simulink model "example1_cs"  (R2018b)
settings: Solver=ode5  StartTime=0.0  StopTime=inf  FixedStep=1/20  RelTol=1e-3
PreLoadFcn:
  | mbxruntime.callbacks.PreLoadFcn(bdroot);
PostLoadFcn:
  | mbxruntime.callbacks.PostLoadFcn(bdroot);
InitFcn:
  | mbxruntime.callbacks.InitFcn(bdroot);
StartFcn:
  | mbxruntime.callbacks.StartFcn(bdroot);
StopFcn:
  | mbxruntime.callbacks.StopFcn(bdroot);
model workspace: external: MAT-File example1_cs_hws.mat (data not in the file)
undefined symbols (not defined in the file or in its folder): Broadcast, CameraTimestamp, Confidence, ConfidenceType, DiscIntNeverNeededParam, ErrorCode, Header, Height, Id, Id_SL_Info, InitImageOutputDir, Length, LidarTimestamp, PerceptionObstacle, PerceptionObstacle_SL_Info, PolygonPoint, PolygonPoint_SL_Info, Pose, Position, RadarTimestamp, S, SequenceNum, Theta, Timestamp, TimestampSec, TrackingTime, Type, Velocity, warningInitialVelocity, Waypoint, Waypoint_SL_Info, Width, X, x0, Y, Z
libraries: simulink x27, robotlib x15, PreScanSimulinkLibrary x14, simulink_extras x5, robotcorelib x2
(part 3 of 5)

== system example1_cs/Ford_Focus_Stationwagon_1 ==
  SELF_Ford_Focus_Stationwagon_1 : Inport  Tag=inport/SelfPort  OutDataTypeStr=Bus: PRESCAN_SELFSENSORDATA  PortDimensions=1  SampleTime=1/20  BusOutputAsStruct=on
  Path : S-Function  Tag=Path  LoadFcn=load('PrescanMotionData.mat')  FunctionName=sfun_Path  Parameters=uniqueID, pathUniqueID, timestep  SFunctionDeploymentMode=off  EnableBusSupport=off  mask(Path){uniqueID=232, pathUniqueID=457, timestep=1/20}
      mask prompts: uniqueID "Object Unique ID"; pathUniqueID "Path Unique ID"; timestep "MATLAB timestep:"
      mask help:
      | The path block outputs the position along a given trajectory.
      |
      | For more information, please click Help.
      mask Help: eval('openHelp(312)')
      mask Display: image(imread('Path.png'))
  SELF_Demux : Subsystem  Tag=demux/SelfPort  mask(PreScan Demux Block:){}
      mask help:
      | The SELF port shows (state) information of the actor itself. The outputs are position in the experiment's axis system and the GPS coordinates, and the object's absolute velocity and compass heading.
      |
      | For more information, please click Help.
      settings: DeleteFcn=PreScanBlockDeleteFcn;
      mask Help: eval('openHelp(462)')
      mask Display:
      | port_label('output',1,'x [m]')
      | port_label('output',2,'y [m]')
      | port_label('output',3,'z [m]','texmode','on')
      | port_label('output',4,'Rotx [deg]','texmode','on')
      | port_label('output',5,'Roty [deg]','texmode','on')
      | port_label('output',6,'Rotz [deg]','texmode','on')
      | port_label('output',7,'GPS lat [deg]','texmode','on')
      | port_label('output',8,'GPS long [deg]','texmode','on')
      | port_label('output',9,'GPS alt [m]','texmode','on')
      | port_label('output',10,'Velocity [m/s]')
      | port_label('output',11,'Heading [deg]')
      | port_label('output',12,'Yaw rate [deg/s]')
  STATE_Ford_Focus_Stationwagon_1_rc : RateTransition  Tag=mux_rc/StatePort  OutPortSampleTimeOpt=Inherit
  SpeedProfile : S-Function  Tag=SpeedProfile  LoadFcn=load('PrescanMotionData.mat')  FunctionName=sfun_SpeedProfile  Parameters=speedProfileUniqueID, timestep  SFunctionDeploymentMode=off  EnableBusSupport=off  mask(SpeedProfile){speedProfileUniqueID=458, timestep=1/20}
      mask prompts: speedProfileUniqueID "Speed Profile Unique ID"; timestep "MATLAB timestep:"
      mask help:
      | The speed profile block outputs the travelled distance, velocities and acceleration along a given path.
      |
      | For more information, please click Help.
      mask Help: eval('openHelp(312)')
      mask Display: image(imread('SpeedProfile.png'))
  Terminator_{1..12} (12 alike) : Terminator
  STATE_Ford_Focus_Stationwagon_1_bus : Outport  Tag=outport/StatePort  OutDataTypeStr=Bus: PRESCAN_STATEACTUATORDATA  PortDimensions=1  SampleTime=1/20
  wires:
  STATE_Ford_Focus_Stationwagon_1_rc/1 -> STATE_Ford_Focus_Stationwagon_1_bus/1
  SpeedProfile/1 -> Path/1
  Path/1 -> STATE_Ford_Focus_Stationwagon_1_rc/1
  SELF_Ford_Focus_Stationwagon_1/1 -> SELF_Demux/1(SELF)
  SELF_Demux/1(x [m]) -> Terminator_1/1
  SELF_Demux/2(y [m]) -> Terminator_2/1
  SELF_Demux/3(z [m]) -> Terminator_3/1
  SELF_Demux/4(rotx [deg]) -> Terminator_4/1
  SELF_Demux/5(roty [deg]) -> Terminator_5/1
  SELF_Demux/6(rotz [deg]) -> Terminator_6/1
  SELF_Demux/7(GPS lat [deg]) -> Terminator_7/1
  SELF_Demux/8(GPS long [deg]) -> Terminator_8/1
  SELF_Demux/9(GPS alt [m]) -> Terminator_9/1
  SELF_Demux/10(velocity [m/s]) -> Terminator_10/1
  SELF_Demux/11(heading [deg]) -> Terminator_11/1
  SELF_Demux/12(yaw rate [deg/s]) -> Terminator_12/1

== system example1_cs/ObjectCameraSensor_1 ==
  Sensor : S-Function  FunctionName=sfun_OCS  Parameters=sensorID, detectableObjects, dataWidth, dataHeight, channelsPerImage, timestep  SFunctionDeploymentMode=off  EnableBusSupport=off  mask(PreScan Source Block: Object Camera Sensor){sensorID=68, detectableObjects=1, dataWidth=240, dataHeight=960, channelsPerImage=3, timestep=1/20}
      mask prompts: sensorID "Sensor ID"; detectableObjects "Max detectable objects:"; dataWidth "Data width"; dataHeight "Data Height"; channelsPerImage "Channels per image"; timestep "MATLAB timestep:"
      mask help: The Object Camera Sensor provides information on objects locations.
      mask Help: eval('openHelp(2401)')
      mask Display: image(imread('ObjectCameraSensorSL.png'))
  ObjectCameraSensor_1 : Outport  Tag=outport/ObjectCamera/data  OutDataTypeStr=Bus: PRESCAN_OCS_MESSAGE  PortDimensions=1  SampleTime=1/20
  ObjectCameraSensor_1_Image : Outport  Tag=outport/ObjectCamera/image  Port=2  OutDataTypeStr=uint8  SampleTime=1/20
  wires:
  Sensor/1 -> ObjectCameraSensor_1/1
  Sensor/2 -> ObjectCameraSensor_1_Image/1

== system example1_cs/PointCloudSensor_1 ==
  Sensor : S-Function  FunctionName=sfun_PCS  Parameters=sensorID, dataWidth, dataHeight, numChannels, dataType, timestep  SFunctionDeploymentMode=off  EnableBusSupport=off  mask(PreScan Source Block: Point Cloud Sensor){sensorID=260, dataWidth=160, dataHeight=960, numChannels=3, dataType=0, timestep=1/20}
      mask prompts: sensorID "Sensor ID"; dataWidth "Data Width"; dataHeight "Data Height"; numChannels "Channel Count"; dataType "Data Type"; timestep "MATLAB timestep:"
      mask help: The Point Cloud Sensor provides XYZ positions relative to the sensor
      mask Help: eval('openHelp(6400)')
      mask Display: image(imread('PointCloudSensorSL.png'))
  PointCloudSensor_1 : Outport  Tag=outport/PointCloudInport  OutDataTypeStr=single  SampleTime=1/20
  wires:
  Sensor/1 -> PointCloudSensor_1/1

== system example1_cs/PreScanTerminator ==
  Terminator : Terminator
  sfun_Terminator : S-Function  FunctionName=sfun_Terminator  Parameters=SampleTime  SFunctionDeploymentMode=off  EnableBusSupport=off  mask(Legacy Function){SFunctionSpec=void prescan_terminator_outputFcn(void ** work1, PRESCAN_TERMINATORDATA y1[1]), SampleTime=TimeStep, ShowSpec=on}
      mask prompts: SampleTime "Sample time (-1 for inherited):"; ShowSpec "Display function specification"
      mask help:
      | This block allows you to call the legacy functions specified by the following Legacy Code Tool definition:
      | def.SFunctionName = 'sfun_Terminator';
      | def.OutputFcnSpec = 'void prescan_terminator_outputFcn(void ** work1, PRESCAN_TERMINATORDATA y1[1])';
      | def.StartFcnSpec = 'void prescan_terminator_startFcn(void ** work1)';
      | def.TerminateFcnSpec = 'void prescan_terminator_terminateFcn(void ** work1)';
      | def.HeaderFiles = {'prescan_terminator_data.h'};
      | def.HostLibFiles = {'sensorinterfaced.lib'};
      | def.IncPaths = {'src', 'C:\prescandev\vislibrary\vis\..\pimp\include\sensors\InterfaceRTW'};
      | def.SrcPaths = {'src'};
      | def.LibPaths = {'C:\\prescandev\\vislibrary_build\lib'};
      | def.SampleTime = 'parameterized';
      | def.Options.language = 'C';
      mask Help: <p>This block was generated automatically by the Legacy Code Tool. For detailed help on this tool, call<a href="matlab:legacy_code('help')"> legacy_code('help')</a>.</p>
      mask Callback ShowSpec:
      | if strcmp(get_param(gcbh, 'ShowSpec'), 'on')
      |   set_param(gcbh, 'MaskDisplay', sprintf('fprintf(''%s'');', get_param(gcbh, 'SFunctionSpec')));
      | else
      |   set_param(gcbh, 'MaskDisplay', sprintf('fprintf(''%s'');', get_param(gcbh, 'FunctionName')));
      | end
      mask Display: fprintf('void prescan_terminator_outputFcn(void ** work1, PRESCAN_TERMINATORDATA y1[1])');
  wires:
  sfun_Terminator/1 -> Terminator/1

== system example1_cs/SELF_BMW_X5_SUV_1 ==
  Sensor : S-Function  FunctionName=sfun_SelfSensor  Parameters=UniqueID, TimeStep  SFunctionDeploymentMode=off  EnableBusSupport=off  mask(PreScan Source Block: SELF){UniqueID=35, TimeStep=1/20}
      mask prompts: UniqueID "Auto-Assigned: Unique ID"; TimeStep "Auto-Assigned: Upload Period [s]"
      mask help:
      | The SELF port shows (state) information of the actor itself. The outputs are position in the experiment's axis system and the GPS coordinates, and the object's absolute velocity and compass heading.
      |
      | For more information, please click Help.
      mask Help: eval('openHelp(462)')
      mask Display: image(imread('GPS.png'))
  SELF_BMW_X5_SUV_1 : Outport  Tag=outport/SelfPort  OutDataTypeStr=Bus: PRESCAN_SELFSENSORDATA  PortDimensions=1  SampleTime=1/20
  wires:
  Sensor/1 -> SELF_BMW_X5_SUV_1/1

== system example1_cs/SELF_Boy_150_1 ==
  Sensor : S-Function  FunctionName=sfun_SelfSensor  Parameters=UniqueID, TimeStep  SFunctionDeploymentMode=off  EnableBusSupport=off  mask(PreScan Source Block: SELF){UniqueID=120, TimeStep=1/20}
      mask prompts: UniqueID "Auto-Assigned: Unique ID"; TimeStep "Auto-Assigned: Upload Period [s]"
      mask help:
      | The SELF port shows (state) information of the actor itself. The outputs are position in the experiment's axis system and the GPS coordinates, and the object's absolute velocity and compass heading.
      |
      | For more information, please click Help.
      mask Help: eval('openHelp(462)')
      mask Display: image(imread('GPS.png'))
  SELF_Boy_150_1 : Outport  Tag=outport/SelfPort  OutDataTypeStr=Bus: PRESCAN_SELFSENSORDATA  PortDimensions=1  SampleTime=1/20
  wires:
  Sensor/1 -> SELF_Boy_150_1/1

== system example1_cs/SELF_Ford_Focus_Stationwagon_1 ==
  Sensor : S-Function  FunctionName=sfun_SelfSensor  Parameters=UniqueID, TimeStep  SFunctionDeploymentMode=off  EnableBusSupport=off  mask(PreScan Source Block: SELF){UniqueID=232, TimeStep=1/20}
      mask prompts: UniqueID "Auto-Assigned: Unique ID"; TimeStep "Auto-Assigned: Upload Period [s]"
      mask help:
      | The SELF port shows (state) information of the actor itself. The outputs are position in the experiment's axis system and the GPS coordinates, and the object's absolute velocity and compass heading.
      |
      | For more information, please click Help.
      mask Help: eval('openHelp(462)')
      mask Display: image(imread('GPS.png'))
  SELF_Ford_Focus_Stationwagon_1 : Outport  Tag=outport/SelfPort  OutDataTypeStr=Bus: PRESCAN_SELFSENSORDATA  PortDimensions=1  SampleTime=1/20
  wires:
  Sensor/1 -> SELF_Ford_Focus_Stationwagon_1/1

== system example1_cs/STATE_BMW_X5_SUV_1_bus ==
  STATE_BMW_X5_SUV_1_bus : Inport  Tag=inport/StatePort  OutDataTypeStr=Bus: PRESCAN_STATEACTUATORDATA  PortDimensions=1  SampleTime=1/20  BusOutputAsStruct=on
  Actuator : S-Function  FunctionName=sfun_StateActuator  Parameters=UniqueID, TimeStep  SFunctionDeploymentMode=off  EnableBusSupport=off  mask(PreScan Sink Block: State){UniqueID=35, TimeStep=1/20}
      mask prompts: UniqueID "Auto-Assigned: Unique ID"; TimeStep "Auto-Assigned: Upload Period [s]"
      mask help:
      | The Actor State contains a vector signal of size (9x1), containing the following signals:
      |
      | -  Position    	(x,y,z)             	[m]
      | -  Velocity    	(vx,vy,vz)         	[m/s]
      | -  Angles       	(Roll, Pitch, Yaw)	[rad]
      |
      | The Actor state is defined in the global axis system.
      | The state is superponed on the Initial position defined in the GUI.
      |
      | For more information, please click Help.
      mask Help: eval('openHelp(222)')
      mask Display: image(imread('State.png'))
  wires:
  STATE_BMW_X5_SUV_1_bus/1 -> Actuator/1

== system example1_cs/STATE_Boy_150_1_bus ==
  STATE_Boy_150_1_bus : Inport  Tag=inport/StatePort  OutDataTypeStr=Bus: PRESCAN_STATEACTUATORDATA  PortDimensions=1  SampleTime=1/20  BusOutputAsStruct=on
  Actuator : S-Function  FunctionName=sfun_StateActuator  Parameters=UniqueID, TimeStep  SFunctionDeploymentMode=off  EnableBusSupport=off  mask(PreScan Sink Block: State){UniqueID=120, TimeStep=1/20}
      mask prompts: UniqueID "Auto-Assigned: Unique ID"; TimeStep "Auto-Assigned: Upload Period [s]"
      mask help:
      | The Actor State contains a vector signal of size (9x1), containing the following signals:
      |
      | -  Position    	(x,y,z)             	[m]
      | -  Velocity    	(vx,vy,vz)         	[m/s]
      | -  Angles       	(Roll, Pitch, Yaw)	[rad]
      |
      | The Actor state is defined in the global axis system.
      | The state is superponed on the Initial position defined in the GUI.
      |
      | For more information, please click Help.
      mask Help: eval('openHelp(222)')
      mask Display: image(imread('State.png'))
  wires:
  STATE_Boy_150_1_bus/1 -> Actuator/1

== system example1_cs/STATE_Ford_Focus_Stationwagon_1_bus ==
  STATE_Ford_Focus_Stationwagon_1_bus : Inport  Tag=inport/StatePort  OutDataTypeStr=Bus: PRESCAN_STATEACTUATORDATA  PortDimensions=1  SampleTime=1/20  BusOutputAsStruct=on
  Actuator : S-Function  FunctionName=sfun_StateActuator  Parameters=UniqueID, TimeStep  SFunctionDeploymentMode=off  EnableBusSupport=off  mask(PreScan Sink Block: State){UniqueID=232, TimeStep=1/20}
      mask prompts: UniqueID "Auto-Assigned: Unique ID"; TimeStep "Auto-Assigned: Upload Period [s]"
      mask help:
      | The Actor State contains a vector signal of size (9x1), containing the following signals:
      |
      | -  Position    	(x,y,z)             	[m]
      | -  Velocity    	(vx,vy,vz)         	[m/s]
      | -  Angles       	(Roll, Pitch, Yaw)	[rad]
      |
      | The Actor state is defined in the global axis system.
      | The state is superponed on the Initial position defined in the GUI.
      |
      | For more information, please click Help.
      mask Help: eval('openHelp(222)')
      mask Display: image(imread('State.png'))
  wires:
  STATE_Ford_Focus_Stationwagon_1_bus/1 -> Actuator/1

== system example1_cs/Synchronizer ==
  Bus Selector1 : BusSelector  OutputSignals=FederateStopped
  Stop Simulation : Stop
  sfun_Synchronizer : S-Function  FunctionName=sfun_Synchronizer  Parameters=SampleTime  SFunctionDeploymentMode=off  EnableBusSupport=off  mask(Legacy Function){SFunctionSpec=void prescan_synchronizer_outputFcn(void ** work1, PRESCAN_SYNCHRONIZEDATA y1[1]), SampleTime=TimeStep, ShowSpec=on}
      mask prompts: SampleTime "Sample time (-1 for inherited):"; ShowSpec "Display function specification"
      mask help:
      | This block allows you to call the legacy functions specified by the following Legacy Code Tool definition:
      | def.SFunctionName = 'sfun_Synchronizer';
      | def.OutputFcnSpec = 'void prescan_synchronizer_outputFcn(void ** work1, PRESCAN_SYNCHRONIZEDATA y1[1])';
      | def.StartFcnSpec = 'void prescan_synchronizer_startFcn(void ** work1)';
      | def.TerminateFcnSpec = 'void prescan_synchronizer_terminateFcn(void ** work1)';
      | def.HeaderFiles = {'prescan_synchronizer_data.h'};
      | def.HostLibFiles = {'sensorinterfaced.lib'};
      | def.IncPaths = {'src', 'C:\prescandev\vislibrary\vis\..\pimp\include\sensors\InterfaceRTW'};
      | def.SrcPaths = {'src'};
      | def.LibPaths = {'C:\\prescandev\\vislibrary_build\lib'};
      | def.SampleTime = 'parameterized';
      | def.Options.language = 'C';
      mask Help: <p>This block was generated automatically by the Legacy Code Tool. For detailed help on this tool, call<a href="matlab:legacy_code('help')"> legacy_code('help')</a>.</p>
      mask Callback ShowSpec:
      | if strcmp(get_param(gcbh, 'ShowSpec'), 'on')
      |   set_param(gcbh, 'MaskDisplay', sprintf('fprintf(''%s'');', get_param(gcbh, 'SFunctionSpec')));
      | else
      |   set_param(gcbh, 'MaskDisplay', sprintf('fprintf(''%s'');', get_param(gcbh, 'FunctionName')));
      | end
      mask Display: fprintf('void prescan_synchronizer_outputFcn(void ** work1, PRESCAN_SYNCHRONIZEDATA y1[1])');
  wires:
  Bus Selector1/1 -> Stop Simulation/1  "<FederateStopped>"
  sfun_Synchronizer/1 -> Bus Selector1/1

== system example1_cs/BMW_X5_SUV_1/BoundingRectangle_1_Demux ==
  BRS : Inport
  Bus Selector : BusSelector  OutputSignals=DATA.ObjectID,DATA.Left,DATA.Right,DATA.Bottom,DATA.Top
  For Iterator : ForIterator  ResetStates=reset  IterationLimit=detectableObjects
  Selector : Selector  InputPortWidth=detectableObjects  IndexOptions=Index vector (port)  Indices=[1 3]  OutputSizes=1
  Signal2ArrayOfSignals1 : Subsystem  mask{VECTORLENGTH=detectableObjects}
      mask prompts: VECTORLENGTH "Length of vector"
  Signal2ArrayOfSignals2 : Subsystem  mask{VECTORLENGTH=detectableObjects}
      mask prompts: VECTORLENGTH "Length of vector"
  Signal2ArrayOfSignals3 : Subsystem  mask{VECTORLENGTH=detectableObjects}
      mask prompts: VECTORLENGTH "Length of vector"
  Signal2ArrayOfSignals4 : Subsystem  mask{VECTORLENGTH=detectableObjects}
      mask prompts: VECTORLENGTH "Length of vector"
  Signal2ArrayOfSignals5 : Subsystem  mask{VECTORLENGTH=detectableObjects}
      mask prompts: VECTORLENGTH "Length of vector"
  ObjectID : Outport
  Left : Outport  Port=2
  Right : Outport  Port=3
  Bottom : Outport  Port=4
  Top : Outport  Port=5
  wires:
  Bus Selector/5 -> Signal2ArrayOfSignals5/2(Element)  "<Top>"
  Signal2ArrayOfSignals5/1(ArrayofElements) -> Top/1
  Bus Selector/4 -> Signal2ArrayOfSignals4/2(Element)  "<Bottom>"
  Signal2ArrayOfSignals4/1(ArrayofElements) -> Bottom/1
  Bus Selector/3 -> Signal2ArrayOfSignals3/2(Element)  "<Right>"
  Signal2ArrayOfSignals3/1(ArrayofElements) -> Right/1
  Bus Selector/2 -> Signal2ArrayOfSignals1/2(Element)  "<Left>"
  Signal2ArrayOfSignals1/1(ArrayofElements) -> Left/1
  Signal2ArrayOfSignals2/1(ArrayofElements) -> ObjectID/1
  Bus Selector/1 -> Signal2ArrayOfSignals2/2(Element)  "<ObjectID>"
  Selector/1 -> Bus Selector/1
  For Iterator/1 -> Signal2ArrayOfSignals4/1(LoopIndex), Signal2ArrayOfSignals5/1(LoopIndex), Signal2ArrayOfSignals3/1(LoopIndex), Signal2ArrayOfSignals1/1(LoopIndex), Signal2ArrayOfSignals2/1(LoopIndex), Selector/2
  BRS/1 -> Selector/1

== system example1_cs/BMW_X5_SUV_1/CameraSensor_1_CM_Demux ==
  In1 : Inport
  Selector : Selector  NumberOfDimensions=2  InputPortWidth=3  IndexOptions=Index vector (dialog),Index vector (dialog)  Indices=-1,1:hres  OutputSizes=1,1
  Selector1 : Selector  NumberOfDimensions=2  InputPortWidth=3  IndexOptions=Index vector (dialog),Index vector (dialog)  Indices=-1,hres+1:hres*2  OutputSizes=1,1
  Selector2 : Selector  NumberOfDimensions=2  InputPortWidth=3  IndexOptions=Index vector (dialog),Index vector (dialog)  Indices=-1,hres*2+1:hres*3  OutputSizes=1,1
  R : Outport
  G : Outport  Port=2
  B : Outport  Port=3
  wires:
  In1/1 -> Selector1/1, Selector/1, Selector2/1
  Selector/1 -> R/1
  Selector1/1 -> G/1
  Selector2/1 -> B/1

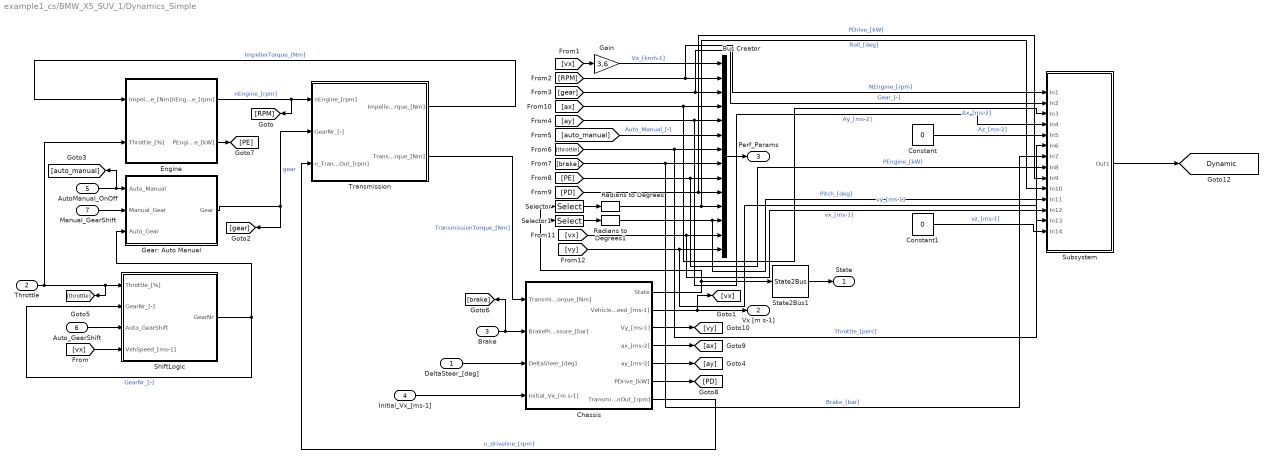
== system example1_cs/BMW_X5_SUV_1/Dynamics_Simple ==
  DeltaSteer_[deg] : Inport
  Throttle : Inport  Port=2
  Brake : Inport  Port=3
  Initial_Vx_[ms-1] : Inport  Port=4
  AutoManual_OnOff : Inport  Port=5
  Auto_GearShift : Inport  Port=6
  Manual_GearShift : Inport  Port=7
  Bus Creator : BusCreator  Inputs=14
  Chassis : Subsystem
      mask Display: image(imread('Chassis.png'));
  Constant : Constant  Value=0
  Constant1 : Constant  Value=0
  Engine : Subsystem
      mask Display: image(imread('Engine.png'));
  Gain : Gain  Gain=3.6
  Gear: Auto Manual : Subsystem
  Radians to Degrees : simulink_extras/Transformations/Radians to Degrees
  Radians to Degrees1 : simulink_extras/Transformations/Radians to Degrees
  Selector : Selector  InputPortWidth=9  IndexOptions=Index vector (dialog)  Indices=7  OutputSizes=1
  Selector1 : Selector  InputPortWidth=9  IndexOptions=Index vector (dialog)  Indices=8  OutputSizes=1
  ShiftLogic : Subsystem
      mask Display: image(imread('Gearshift.png'));
  State2Bus1 : PreScanSimulinkLibrary/State2Bus  Tag=State  Priority=0  x0=initialX  y0=initialY  z0=initialZ  Roll0=initialRoll  Pitch0=initialPitch  Yaw0=initialYaw  TimeStep=TimeStep
  Subsystem : Subsystem
  Transmission : Subsystem
      mask Display: image(imread('Transmission.png'));
  State : Outport
  Vx [m s-1] : Outport  Port=2
  Perf_Params : Outport  Port=3
  tag scope: Dynamic=global
  wires:
  State2Bus1/1 -> State/1
  [vy] -> Subsystem/13(In13), Bus Creator/14  "vy_[ms-1]"
  [vx] -> Subsystem/12(In12), Bus Creator/13  "vx_[ms-1]"
  Chassis/7(TransmissionOut_[rpm]) -> Transmission/3(n_TransmissionOut_[rpm])  "n_driveline_[rpm]"
  Chassis/6(PDrive_[kW]) -> [PD]
  Chassis/5(ay_[ms-2]) -> [ay]
  Chassis/4(ax_[ms-2]) -> [ax]
  Chassis/3(Vy_[ms-1]) -> [vy]
  [vx] -> ShiftLogic/4(VehSpeed_[ms-1])
  Gear: Auto Manual/1(Gear) -> Transmission/2(GearNr_[-]), [gear]  "gear"
  Manual_GearShift/1 -> Gear: Auto Manual/2(Manual_Gear)
  AutoManual_OnOff/1 -> Gear: Auto Manual/1(Auto_Manual), [auto_manual]
  Chassis/2(VehicleSpeed_[ms-1]) -> [vx], Vx [m s-1]/1
  Auto_GearShift/1 -> ShiftLogic/3(Auto_GearShift)
  Throttle/1 -> Engine/2(Throttle_[%]), ShiftLogic/1(Throttle_[%]), [throttle]
  Initial_Vx_[ms-1]/1 -> Chassis/4(Initial_Vx_[m s-1])
  DeltaSteer_[deg]/1 -> Chassis/3(DeltaSteer_[deg])
  Chassis/1(State) -> Selector/1, Selector1/1, State2Bus1/1
  Brake/1 -> [brake], Chassis/2(BrakePressure_[bar])
  Engine/1(nEngine_[rpm]) -> [RPM], Transmission/1(nEngine_[rpm])  "nEngine_[rpm]"
  ShiftLogic/1(GearNr) -> Gear: Auto Manual/3(Auto_Gear), ShiftLogic/2(GearNr_[-])  "GearNr_[-]"
  Transmission/2(TransmissionTorque_[Nm]) -> Chassis/1(TransmissionTorque_[Nm])  "TransmissionTorque_[Nm]"
  Transmission/1(ImpellerTorque_[Nm]) -> Engine/1(ImpellerTorque_[Nm])  "ImpellerTorque_[Nm]"
  Gain/1 -> Bus Creator/1  "Vx_[kmh-1]"
  [RPM] -> Subsystem/1(In1), Bus Creator/2  "NEngine_[rpm]"
  [gear] -> Subsystem/2(In2), Bus Creator/3  "Gear_[-]"
  [ay] -> Subsystem/4(In4), Bus Creator/5  "Ay_[ms-2]"
  [auto_manual] -> Bus Creator/6  "Auto_Manual_[-]"
  [throttle] -> Subsystem/6(In6), Bus Creator/7  "Throttle_[perc]"
  [brake] -> Subsystem/7(In7), Bus Creator/8  "Brake_[bar]"
  Engine/2(PEngine_[kW]) -> [PE]
  Bus Creator/1 -> Perf_Params/1
  [PE] -> Subsystem/8(In8), Bus Creator/9  "PEngine_[kW]"
  Radians to Degrees/1 -> Subsystem/10(In10), Bus Creator/11  "Roll_[deg]"
  Radians to Degrees1/1 -> Subsystem/11(In11), Bus Creator/12  "Pitch_[deg]"
  [PD] -> Subsystem/9(In9), Bus Creator/10  "PDrive_[kW]"
  Selector/1 -> Radians to Degrees/1
  Selector1/1 -> Radians to Degrees1/1
  [vx] -> Gain/1
  [ax] -> Subsystem/3(In3), Bus Creator/4  "Ax_[ms-2]"
  Constant/1 -> Subsystem/5(In5)  "Az_[ms-2]"
  Constant1/1 -> Subsystem/14(In14)  "vz_[ms-1]"
  Subsystem/1(Out1) -> [Dynamic]

== system example1_cs/BMW_X5_SUV_1/Enabled Subsystem ==
  In1 : Inport
  Enable : EnablePort
  Add : Sum
  Bus Selector : BusSelector  DialogController=Simulink.DDGSource_BusSelector  OutputSignals=Throttle,Brake,Debug.SimpleLatDebug.SteerAngle,Debug.SimpleLatDebug.RefSpeed,Debug.InputDebug.LocalizationHeader.TimestampSec
  Display : Display
  Ground_1 : Ground
  Product : Product
  Step : Step  Time=5  After=-30  SampleTime=0
  Step1 : Step  Time=5  Before=1  After=0  SampleTime=0
  Terminator_1 : Terminator
  Out1 : Outport
  Out2 : Outport  Port=2
  Out3 : Outport  Port=3
  Out5 : Outport  Port=4
  Out4 : Outport  Port=5
  wires:
  In1/1 -> Bus Selector/1
  Bus Selector/1 -> Out1/1  "<Throttle>"
  Bus Selector/2 -> Out2/1  "<Brake>"
  Bus Selector/4 -> Out5/1  "<RefSpeed>"
  Step/1 -> Add/1
  Step1/1 -> Product/2
  Product/1 -> Add/2
  Bus Selector/3 -> Out3/1, Display/1  "<SteerAngle>"
  Bus Selector/5 -> Out4/1  "<TimestampSec>"
  Add/1 -> Terminator_1/1
  Ground_1/1 -> Product/1

== system example1_cs/BMW_X5_SUV_1/Enabled Subsystem1 ==
  In1 : Inport
  Enable : EnablePort
  Add : Sum
  Bus Selector : BusSelector  DialogController=Simulink.DDGSource_BusSelector  OutputSignals=TrajectoryPoint,TrajectoryPoint_SL_Info
  Ground_1 : Ground
  Product : Product
  Step : Step  Time=5  After=-30  SampleTime=0
  Step1 : Step  Time=5  Before=1  After=0  SampleTime=0
  Terminator_1 : Terminator
  Out1 : Outport
  Out2 : Outport  Port=2
  wires:
  In1/1 -> Bus Selector/1
  Bus Selector/1 -> Out1/1  "<TrajectoryPoint>"
  Bus Selector/2 -> Out2/1  "<TrajectoryPoint_SL_Info>"
  Step/1 -> Add/1
  Step1/1 -> Product/2
  Product/1 -> Add/2
  Add/1 -> Terminator_1/1
  Ground_1/1 -> Product/1

== system example1_cs/BMW_X5_SUV_1/ObjectCameraSensor_1_Demux ==
  OCS : Inport
  Bus Creator1 : BusCreator  Inputs=16
  Bus Selector : BusSelector  OutputSignals=DATA.ObjectID,DATA.ObjectTypeID,DATA.Left,DATA.Right,DATA.Bottom,DATA.Top,DATA.Range,DATA.DopplerVelocity,DATA.Theta,DATA.Phi
  For Iterator : ForIterator  ResetStates=reset  IterationLimit=detectableObjects
  Selector : Selector  InputPortWidth=detectableObjects  IndexOptions=Index vector (port)  Indices=[1 3]  OutputSizes=1
  Signal2ArrayOfSignals1 : PreScanSimulinkLibrary/DemuxBRS/Signal2ArrayOfSignals1  VECTORLENGTH=detectableObjects
  Signal2ArrayOfSignals{5,7..10} (5 alike) : PreScanSimulinkLibrary/DemuxBRS/Signal2ArrayOfSignals5  VECTORLENGTH=detectableObjects
  Signal2ArrayOfSignals2 : PreScanSimulinkLibrary/DemuxBRS/Signal2ArrayOfSignals2  VECTORLENGTH=detectableObjects
  Signal2ArrayOfSignals3 : PreScanSimulinkLibrary/DemuxBRS/Signal2ArrayOfSignals3  VECTORLENGTH=detectableObjects
  Signal2ArrayOfSignals4 : PreScanSimulinkLibrary/DemuxBRS/Signal2ArrayOfSignals4  VECTORLENGTH=detectableObjects
  Signal2ArrayOfSignals6 : PreScanSimulinkLibrary/DemuxBRS/Signal2ArrayOfSignals1  VECTORLENGTH=detectableObjects
  ToCamAxesComponents1 : Subsystem
  ToCamAxesComponents2 : Subsystem
  OCS Data : Outport
  wires:
  OCS/1 -> Selector/1
  For Iterator/1 -> Selector/2, Signal2ArrayOfSignals2/1, Signal2ArrayOfSignals1/1, Signal2ArrayOfSignals3/1, Signal2ArrayOfSignals5/1, Signal2ArrayOfSignals4/1, Signal2ArrayOfSignals6/1, Signal2ArrayOfSignals7/1, Signal2ArrayOfSignals8/1, Signal2ArrayOfSignals9/1, Signal2ArrayOfSignals10/1
  Selector/1 -> Bus Selector/1
  Bus Selector/1 -> Signal2ArrayOfSignals2/2  "<ObjectID>"
  Bus Selector/3 -> Signal2ArrayOfSignals1/2  "<Left>"
  Bus Selector/4 -> Signal2ArrayOfSignals3/2  "<Right>"
  Bus Selector/5 -> Signal2ArrayOfSignals4/2  "<Bottom>"
  Bus Selector/6 -> Signal2ArrayOfSignals5/2  "<Top>"
  Signal2ArrayOfSignals2/1 -> Bus Creator1/1  "Object ID[-]"
  Signal2ArrayOfSignals1/1 -> Bus Creator1/3  "Left[-]"
  Signal2ArrayOfSignals6/1 -> Bus Creator1/2  "ObjectTypeID[-]"
  Signal2ArrayOfSignals3/1 -> Bus Creator1/4  "Right[-]"
  Bus Creator1/1 -> OCS Data/1  "OCS Data"
  Signal2ArrayOfSignals7/1 -> ToCamAxesComponents1/1(rho), Bus Creator1/7  "Range[m]"
  ToCamAxesComponents1/1(ComponentX) -> Bus Creator1/8  "RangeX[m]"
  ToCamAxesComponents1/2(ComponentY) -> Bus Creator1/9  "RangeY[m]"
  ToCamAxesComponents1/3(ComponentZ) -> Bus Creator1/10  "RangeZ[m]"
  ToCamAxesComponents2/1(ComponentX) -> Bus Creator1/12  "DopplerVelocityX[ms-1]"
  ToCamAxesComponents2/2(ComponentY) -> Bus Creator1/13  "DopplerVelocityY[ms-1]"
  ToCamAxesComponents2/3(ComponentZ) -> Bus Creator1/14  "DopplerVelocityZ[ms-1]"
  Signal2ArrayOfSignals9/1 -> Bus Creator1/15, ToCamAxesComponents2/2(theta), ToCamAxesComponents1/2(theta)  "Theta[deg]"
  Signal2ArrayOfSignals10/1 -> Bus Creator1/16, ToCamAxesComponents2/3(phi), ToCamAxesComponents1/3(phi)  "Phi[deg]"
  Bus Selector/2 -> Signal2ArrayOfSignals6/2  "<ObjectTypeID>"
  Bus Selector/7 -> Signal2ArrayOfSignals7/2  "<Range>"
  Bus Selector/8 -> Signal2ArrayOfSignals8/2  "<DopplerVelocity>"
  Bus Selector/9 -> Signal2ArrayOfSignals9/2  "<Theta>"
  Bus Selector/10 -> Signal2ArrayOfSignals10/2  "<Phi>"
  Signal2ArrayOfSignals8/1 -> ToCamAxesComponents2/1(rho), Bus Creator1/11  "DopplerVelocity[ms-1]"
  Signal2ArrayOfSignals4/1 -> Bus Creator1/5  "Bottom[-]"
  Signal2ArrayOfSignals5/1 -> Bus Creator1/6  "Top[-]"

== system example1_cs/BMW_X5_SUV_1/ObjectCameraSensor_1_Image_Demux ==
  In1 : Inport
  Selector : Selector  NumberOfDimensions=2  InputPortWidth=3  IndexOptions=Index vector (dialog),Index vector (dialog)  Indices=-1,1:hres  OutputSizes=1,1
  Selector1 : Selector  NumberOfDimensions=2  InputPortWidth=3  IndexOptions=Index vector (dialog),Index vector (dialog)  Indices=-1,hres+1:hres*2  OutputSizes=1,1
  Selector2 : Selector  NumberOfDimensions=2  InputPortWidth=3  IndexOptions=Index vector (dialog),Index vector (dialog)  Indices=-1,hres*2+1:hres*3  OutputSizes=1,1
  R : Outport
  G : Outport  Port=2
  B : Outport  Port=3
  wires:
  In1/1 -> Selector1/1, Selector/1, Selector2/1
  Selector/1 -> R/1
  Selector1/1 -> G/1
  Selector2/1 -> B/1

== system example1_cs/BMW_X5_SUV_1/PathFollower_Preview_1 ==
  ActorOffset_Left(+) / Right(-) [m] : Inport
  position x,y,Y [m,m,deg] : Inport  Port=2
  Initial Velocity [m/s] : Inport  Port=3
  Desired Velocity [m/s] : Inport  Port=4
  velocity [m/s] : Inport  Port=5
  vx [m/s] : Inport  Port=6
  vy [m/s] : Inport  Port=7
  Yaw rate [deg/s] : Inport  Port=8
  CorneringStiffness_Tyres_Front [N/rad] : Inport  Port=9
  CorneringStiffness_Tyres_Rear [N/rad] : Inport  Port=10
  steering_ratio[-] : Inport  Port=11
  LateralController : Subsystem
  LongitudinalController : Subsystem
  delta_steerwheel [deg] : Outport
  throttle [%] : Outport  Port=2
  brake pressure [bar] : Outport  Port=3
  v0 [m/s] : Outport  Port=4
  Auto_GearShift : Outport  Port=5
  Actor/Traj_distance [m] : Outport  Port=6
  Actor/Traj_angle [deg] : Outport  Port=7
  wires:
  LateralController/3(delta_steerwheel [deg]) -> delta_steerwheel [deg]/1
  steering_ratio[-]/1 -> LateralController/8(steering_ratio[-])
  CorneringStiffness_Tyres_Rear [N/rad]/1 -> LateralController/7(CorneringStiffness_Tyres_Rear [N/rad])
  CorneringStiffness_Tyres_Front [N/rad]/1 -> LateralController/6(CorneringStiffness_Tyres_Front [N/rad])
  Yaw rate [deg/s]/1 -> LateralController/5(Yaw rate [deg/s])
  vy [m/s]/1 -> LateralController/4(vy [m/s])
  vx [m/s]/1 -> LateralController/3(vx [m/s])
  position x,y,Y [m,m,deg]/1 -> LateralController/2(position x,y,Y [m,m,deg])
  ActorOffset_Left(+) / Right(-) [m]/1 -> LateralController/1(ActorOffset_Left(+) / Right(-) [m])
  LateralController/2(Actor/Traj_angle [deg]) -> Actor/Traj_angle [deg]/1
  LateralController/1(Actor/Traj_distance [m]) -> Actor/Traj_distance [m]/1
  velocity [m/s]/1 -> LongitudinalController/1(v_actual [m/s])
  LongitudinalController/1(throttle [%]) -> throttle [%]/1
  Desired Velocity [m/s]/1 -> LongitudinalController/2(Desired Velocity [m/s])
  Initial Velocity [m/s]/1 -> LongitudinalController/3(Initial Velocity [m/s])
  LongitudinalController/2(brake pressure [bar]) -> brake pressure [bar]/1
  LongitudinalController/3(v0 [m/s]) -> v0 [m/s]/1
  LongitudinalController/4(Auto_GearShift) -> Auto_GearShift/1

== system example1_cs/BMW_X5_SUV_1/PointCloudSensor_1_WorldPos_Demux ==
  In1 : Inport
  Selector : Selector  NumberOfDimensions=2  InputPortWidth=3  IndexOptions=Index vector (dialog),Index vector (dialog)  Indices=-1,offset+1:(offset+hres)  OutputSizes=1,1
  Selector1 : Selector  NumberOfDimensions=2  InputPortWidth=3  IndexOptions=Index vector (dialog),Index vector (dialog)  Indices=-1,(offset+hres+1):(offset+2*hres)  OutputSizes=1,1
  Selector2 : Selector  NumberOfDimensions=2  InputPortWidth=3  IndexOptions=Index vector (dialog),Index vector (dialog)  Indices=-1,(offset+2*hres+1):(offset+3*hres)  OutputSizes=1,1
  X : Outport
  Y : Outport  Port=2
  Z : Outport  Port=3
  wires:
  Selector2/1 -> Z/1
  Selector1/1 -> Y/1
  Selector/1 -> X/1
  In1/1 -> Selector2/1, Selector/1, Selector1/1

== system example1_cs/BMW_X5_SUV_1/SELF_Demux ==
  SELF : Inport  OutDataTypeStr=Bus: PRESCAN_SELFSENSORDATA
  Bus Selector : BusSelector  OutputSignals=PositionX,PositionY,PositionZ,OrientationRoll,OrientationPitch,OrientationYaw,Velocity,Yaw_rate,Lat,Long,Alt
  Demux2 : Demux  Outputs=3
  Gain : Gain  Gain=180/pi
  Gain1 : Gain  Gain=180/pi
  Vector Concatenate1 : Concatenate  NumInputs=3
  compas converter : Subsystem
  x [m] : Outport
  y [m] : Outport  Port=2
  z [m] : Outport  Port=3
  rotx [deg] : Outport  Port=4
  roty [deg] : Outport  Port=5
  rotz [deg] : Outport  Port=6
  GPS lat [deg] : Outport  Port=7
  GPS long [deg] : Outport  Port=8
  GPS alt [m] : Outport  Port=9
  velocity [m/s] : Outport  Port=10
  heading [deg] : Outport  Port=11
  yaw rate [deg/s] : Outport  Port=12
  wires:
  Bus Selector/11 -> GPS alt [m]/1  "<Alt>"
  Bus Selector/10 -> GPS long [deg]/1  "<Long>"
  Bus Selector/9 -> GPS lat [deg]/1  "<Lat>"
  Bus Selector/8 -> Gain1/1  "<Yaw_rate>"
  Bus Selector/7 -> velocity [m/s]/1  "<Velocity>"
  Bus Selector/6 -> compas converter/1(rotz [rad]), Vector Concatenate1/3  "<OrientationYaw>"
  Bus Selector/5 -> Vector Concatenate1/2  "<OrientationPitch>"
  Bus Selector/4 -> Vector Concatenate1/1  "<OrientationRoll>"
  Vector Concatenate1/1 -> Gain/1
  Bus Selector/3 -> z [m]/1  "<PositionZ>"
  Bus Selector/2 -> y [m]/1  "<PositionY>"
  Bus Selector/1 -> x [m]/1  "<PositionX>"
  SELF/1 -> Bus Selector/1
  Gain/1 -> Demux2/1
  Demux2/1 -> rotx [deg]/1
  Demux2/2 -> roty [deg]/1
  Demux2/3 -> rotz [deg]/1
  compas converter/1(heading [deg]) -> heading [deg]/1
  Gain1/1 -> yaw rate [deg/s]/1

== system example1_cs/BMW_X5_SUV_1/State2PathFollowerCnv ==
  State BUS : Inport  OutDataTypeStr=Bus: PRESCAN_STATEACTUATORDATA
  Bus Selector : BusSelector  OutputSignals=AngularVelocityYaw,VelocityX,VelocityY,PositionX,PositionY,OrientationYaw
  Radians to Degrees : simulink_extras/Transformations/Radians to Degrees
  Radians to Degrees1 : simulink_extras/Transformations/Radians to Degrees
  SELF2PathFollowerMux : Mux  Tag=SELF2PathFollowerMux  Inputs=3
  velocity magnitude : Math  Operator=hypot  SaturateOnIntegerOverflow=on
  Yaw rate [deg/s] : Outport
  velocity [m/s] : Outport  Port=2
  position x,y,Y [m,m,deg] : Outport  Port=3
  wires:
  Radians to Degrees1/1 -> Yaw rate [deg/s]/1
  Bus Selector/1 -> Radians to Degrees1/1  "<AngularVelocityYaw>"
  velocity magnitude/1 -> velocity [m/s]/1
  SELF2PathFollowerMux/1 -> position x,y,Y [m,m,deg]/1
  State BUS/1 -> Bus Selector/1
  Bus Selector/2 -> velocity magnitude/1  "<VelocityX>"
  Bus Selector/3 -> velocity magnitude/2  "<VelocityY>"
  Radians to Degrees/1 -> SELF2PathFollowerMux/3
  Bus Selector/6 -> Radians to Degrees/1  "<OrientationYaw>"
  Bus Selector/4 -> SELF2PathFollowerMux/1  "<PositionX>"
  Bus Selector/5 -> SELF2PathFollowerMux/2  "<PositionY>"

== system example1_cs/BMW_X5_SUV_1/Subsystem ==
  In1 : Inport
  In2 : Inport  Port=2
  In3 : Inport  Port=3
  In4 : Inport  Port=4
  In5 : Inport  Port=5
  In6 : Inport  Port=6
  In7 : Inport  Port=7
  In8 : Inport  Port=8
  In9 : Inport  Port=9
  In10 : Inport  Port=10
  In11 : Inport  Port=11
  In12 : Inport  Port=12
  In13 : Inport  Port=13
  Bus Creator : BusCreator  Inputs=13
  Out1 : Outport
  wires:
  In6/1 -> Bus Creator/6
  In5/1 -> Bus Creator/5
  In4/1 -> Bus Creator/4
  In3/1 -> Bus Creator/3
  In2/1 -> Bus Creator/2
  In1/1 -> Bus Creator/1
  In7/1 -> Bus Creator/7
  In8/1 -> Bus Creator/8
  In9/1 -> Bus Creator/9
  In10/1 -> Bus Creator/10
  In11/1 -> Bus Creator/11
  Bus Creator/1 -> Out1/1
  In12/1 -> Bus Creator/12
  In13/1 -> Bus Creator/13

== system example1_cs/BMW_X5_SUV_1/Subsystem1 ==
  In1 : Inport
  In2 : Inport  Port=2
  In3 : Inport  Port=3
  In4 : Inport  Port=4
  In5 : Inport  Port=5
  Bus Creator : BusCreator  Inputs=5
  Out1 : Outport
  wires:
  In5/1 -> Bus Creator/5
  In4/1 -> Bus Creator/4
  In3/1 -> Bus Creator/3
  In2/1 -> Bus Creator/2
  In1/1 -> Bus Creator/1
  Bus Creator/1 -> Out1/1

== system example1_cs/BMW_X5_SUV_1/Subsystem10 ==
  Constant : Constant  Value=5  SampleTime=0.05
  Constant1 : Constant  Value=100
  Constant2 : Constant  Value=5
  Digital Clock : DigitalClock
  Display{1..6,8} (7 alike) : Display
  Divide : Product  Inputs=*/
  Divide1 : Product  Inputs=*/
  If : If  IfExpression=(u1 == 0)
  If Action Subsystem : Subsystem  TreatAsAtomicUnit=on
  Math Function : Math  Operator=rem  SaturateOnIntegerOverflow=on
  Ramp : simulink/Sources/Ramp  slope=0.01  start=0  InitialOutput=0
  Terminator_1 : Terminator
  Out1 : Outport
  Out2 : Outport  Port=2
  Out3 : Outport  Port=3
  wires:
  If/1 -> If Action Subsystem/Action
  Divide/1 -> Out1/1, Display4/1  "timestamp"
  Constant1/1 -> Divide/2
  Divide1/1 -> Display2/1  "sequence"
  If Action Subsystem/1(Out1) -> Divide1/1, Divide/1, Display1/1
  Math Function/1 -> If/1, Display6/1
  Constant2/1 -> Divide1/2
  Constant/1 -> Math Function/2
  Digital Clock/1 -> Out3/1, Display3/1
  Ramp/1 -> Out2/1, Display8/1, If Action Subsystem/1(In1), Math Function/1, Display5/1
  If/2 -> Terminator_1/1

== system example1_cs/BMW_X5_SUV_1/Subsystem11 ==
  In1 : Inport
  Constant14 : Constant
  If : If
  If Action Subsystem : Subsystem  TreatAsAtomicUnit=on
  If Action Subsystem1 : Subsystem  TreatAsAtomicUnit=on
  Merge : Merge
  Out1 : Outport
  wires:
  If Action Subsystem/1(Out1) -> Merge/1
  In1/1 -> If Action Subsystem/1(In1), If/1
  If/2 -> If Action Subsystem1/Action
  If/1 -> If Action Subsystem/Action
  If Action Subsystem1/1(Out1) -> Merge/2
  Constant14/1 -> If Action Subsystem1/1(In1)
  Merge/1 -> Out1/1

== system example1_cs/BMW_X5_SUV_1/Subsystem12 ==
  In1 : Inport
  Constant14 : Constant
  If : If
  If Action Subsystem : Subsystem  TreatAsAtomicUnit=on
  If Action Subsystem1 : Subsystem  TreatAsAtomicUnit=on
  Merge : Merge
  Out1 : Outport
  wires:
  If Action Subsystem/1(Out1) -> Merge/1
  In1/1 -> If Action Subsystem/1(In1), If/1
  If/2 -> If Action Subsystem1/Action
  If/1 -> If Action Subsystem/Action
  If Action Subsystem1/1(Out1) -> Merge/2
  Constant14/1 -> If Action Subsystem1/1(In1)
  Merge/1 -> Out1/1

== system example1_cs/BMW_X5_SUV_1/Subsystem13 ==
  Steering Rate : Inport
  Constant21 : Constant
  Divide3 : Product  Inputs=**
  Unary Minus : UnaryMinus
  Out1 : Outport
  wires:
  Steering Rate/1 -> Divide3/1
  Constant21/1 -> Divide3/2
  Divide3/1 -> Out1/1

== system example1_cs/BMW_X5_SUV_1/Subsystem14 ==
  Throttle : Inport
  Constant19 : Constant  Value=100
  Constant20 : Constant  Value=100
  Divide2 : Product  Inputs=**/
  Out1 : Outport
  wires:
  Divide2/1 -> Out1/1
  Throttle/1 -> Divide2/1
  Constant19/1 -> Divide2/2
  Constant20/1 -> Divide2/3

== system example1_cs/BMW_X5_SUV_1/Subsystem15 ==
  Throttle : Inport
  Constant19 : Constant  Value=0.91
  Divide2 : Product  Inputs=**
  Out1 : Outport
  wires:
  Divide2/1 -> Out1/1
  Throttle/1 -> Divide2/1
  Constant19/1 -> Divide2/2

== system example1_cs/BMW_X5_SUV_1/Subsystem16 ==
  In1 : Inport
  Constant14 : Constant  Value=0
  If : If  IfExpression=-5<u1<5
  If Action Subsystem : Subsystem  TreatAsAtomicUnit=on
  If Action Subsystem1 : Subsystem  TreatAsAtomicUnit=on
  Merge : Merge
  Out1 : Outport
  wires:
  If Action Subsystem/1(Out1) -> Merge/1
  In1/1 -> If Action Subsystem1/1(In1), If/1
  If/2 -> If Action Subsystem1/Action
  If/1 -> If Action Subsystem/Action
  If Action Subsystem1/1(Out1) -> Merge/2
  Merge/1 -> Out1/1
  Constant14/1 -> If Action Subsystem/1(In1)

== system example1_cs/BMW_X5_SUV_1/Subsystem2 ==
  Blank Message21 : robotlib/Blank Message  messageClass=Message  entityType=my_msgs/LaneWayPoint  messageType=my_msgs/LaneWayPoint  SampleTime=inf
      settings: SourceProductBaseCode=RO
  String Constant : StringConstant  String="\"lane_40\""
  String Length : StringLength
  String to ASCII : StringToASCII  MaximumLength=128
  Out1 : Outport
  Out2 : Outport  Port=2
  Out3 : Outport  Port=3
  wires:
  String Length/1 -> Out3/1
  Blank Message21/1 -> Out1/1
  String to ASCII/1 -> Out2/1
  String Constant/1 -> String to ASCII/1, String Length/1

== system example1_cs/BMW_X5_SUV_1/Subsystem3 ==
  Constant353 : Constant  Value=9.9
  Constant354 : Constant  Value=6.6
  Constant355 : Constant  Value=5
  Constant356 : Constant  Value=8.8
  Constant357 : Constant
  Constant359 : Constant
  Constant365 : Constant  Value=6.6
  Data Type Conversion96 : DataTypeConversion
  Data Type Conversion98 : DataTypeConversion
  Data Type Conversion99 : DataTypeConversion
  Out1 : Outport
  Out2 : Outport  Port=2
  Out3 : Outport  Port=3
  Out4 : Outport  Port=4
  Out5 : Outport  Port=5
  Out6 : Outport  Port=6
  Out7 : Outport  Port=7
  wires:
  Data Type Conversion99/1 -> Out7/1
  Constant359/1 -> Data Type Conversion99/1
  Data Type Conversion98/1 -> Out3/1
  Data Type Conversion96/1 -> Out6/1
  Constant354/1 -> Out2/1
  Constant356/1 -> Out4/1
  Constant353/1 -> Out5/1
  Constant355/1 -> Data Type Conversion98/1
  Constant365/1 -> Out1/1
  Constant357/1 -> Data Type Conversion96/1

== system example1_cs/BMW_X5_SUV_1/Subsystem4 ==
  Blank Message21 : robotlib/Blank Message  messageClass=Message  entityType=my_msgs/LaneWayPoint  messageType=my_msgs/LaneWayPoint  SampleTime=inf
      settings: SourceProductBaseCode=RO
  String Constant : StringConstant  String="\"lane_38\""
  String Length : StringLength
  String to ASCII : StringToASCII  MaximumLength=128
  Out1 : Outport
  Out2 : Outport  Port=2
  Out3 : Outport  Port=3
  wires:
  String Length/1 -> Out3/1
  Blank Message21/1 -> Out1/1
  String to ASCII/1 -> Out2/1
  String Constant/1 -> String to ASCII/1, String Length/1

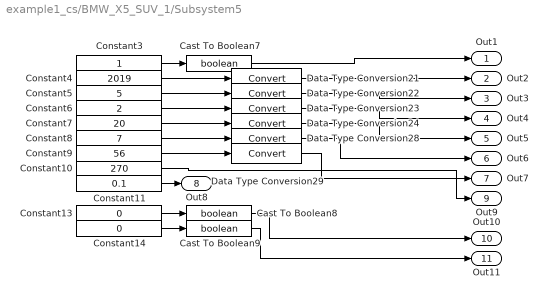
== system example1_cs/BMW_X5_SUV_1/Subsystem5 ==
  Cast To Boolean7 : DataTypeConversion  OutDataTypeStr=boolean
  Cast To Boolean8 : DataTypeConversion  OutDataTypeStr=boolean
  Cast To Boolean9 : DataTypeConversion  OutDataTypeStr=boolean
  Constant10 : Constant  Value=270
  Constant11 : Constant  Value=0.1
  Constant13 : Constant  Value=0
  Constant14 : Constant  Value=0
  Constant3 : Constant
  Constant4 : Constant  Value=2019
  Constant5 : Constant  Value=5
  Constant6 : Constant  Value=2
  Constant7 : Constant  Value=20
  Constant8 : Constant  Value=7
  Constant9 : Constant  Value=56
  Data Type Conversion{21..24,28..29} (6 alike) : DataTypeConversion
  Out1 : Outport
  Out2 : Outport  Port=2
  Out3 : Outport  Port=3
  Out4 : Outport  Port=4
  Out5 : Outport  Port=5
  Out6 : Outport  Port=6
  Out7 : Outport  Port=7
  Out8 : Outport  Port=8
  Out9 : Outport  Port=9
  Out10 : Outport  Port=10
  Out11 : Outport  Port=11
  wires:
  Constant3/1 -> Cast To Boolean7/1
  Constant13/1 -> Cast To Boolean8/1
  Constant14/1 -> Cast To Boolean9/1
  Constant9/1 -> Data Type Conversion29/1
  Data Type Conversion28/1 -> Out6/1
  Cast To Boolean8/1 -> Out10/1
  Cast To Boolean7/1 -> Out1/1
  Constant11/1 -> Out8/1
  Data Type Conversion29/1 -> Out7/1
  Data Type Conversion23/1 -> Out4/1
  Data Type Conversion24/1 -> Out5/1
  Constant7/1 -> Data Type Conversion24/1
  Constant8/1 -> Data Type Conversion28/1
  Data Type Conversion21/1 -> Out2/1
  Data Type Conversion22/1 -> Out3/1
  Constant10/1 -> Out9/1
  Cast To Boolean9/1 -> Out11/1
  Constant5/1 -> Data Type Conversion22/1
  Constant6/1 -> Data Type Conversion23/1
  Constant4/1 -> Data Type Conversion21/1

== system example1_cs/BMW_X5_SUV_1/Subsystem6 ==
  Constant12 : Constant  Value=15
  Data Type Conversion30 : DataTypeConversion
  Out1 : Outport
  wires:
  Data Type Conversion30/1 -> Out1/1
  Constant12/1 -> Data Type Conversion30/1

== system example1_cs/BMW_X5_SUV_1/Subsystem7 ==
  Cast To Boolean{1..6} (6 alike) : DataTypeConversion  OutDataTypeStr=boolean
  Complete_auto_drive : Constant
  Constant2 : Constant  Value=0
  Data Type Conversion3 : DataTypeConversion
  Out1 : Outport
  Out2 : Outport  Port=2
  Out3 : Outport  Port=3
  Out4 : Outport  Port=4
  Out5 : Outport  Port=5
  Out6 : Outport  Port=6
  Out7 : Outport  Port=7
  wires:
  Cast To Boolean3/1 -> Out3/1
  Constant2/1 -> Cast To Boolean6/1, Cast To Boolean5/1, Cast To Boolean4/1, Cast To Boolean3/1, Cast To Boolean2/1, Cast To Boolean1/1
  Complete_auto_drive/1 -> Data Type Conversion3/1
  Cast To Boolean1/1 -> Out1/1
  Cast To Boolean5/1 -> Out5/1
  Data Type Conversion3/1 -> Out7/1
  Cast To Boolean2/1 -> Out2/1
  Cast To Boolean6/1 -> Out6/1
  Cast To Boolean4/1 -> Out4/1

== system example1_cs/BMW_X5_SUV_1/Subsystem8 ==
  Cast To Boolean : DataTypeConversion  OutDataTypeStr=boolean
  Constant42 : Constant
  Out1 : Outport
  wires:
  Constant42/1 -> Cast To Boolean/1
  Cast To Boolean/1 -> Out1/1

== system example1_cs/BMW_X5_SUV_1/Subsystem9 ==
  " " : DataTypeConversion
  Constant1 : Constant  Value=0
  Out1 : Outport
  Out2 : Outport  Port=2
  wires:
  Constant1/1 -> Out1/1, " "/1
  " "/1 -> Out2/1

== system example1_cs/Boy_150_1/Animation ==
  In1 : Inport
  Bus Creator : BusCreator  Inputs=2  OutDataTypeStr=Bus: PRESCAN_ANIMACTUATORDATA  NonVirtualBus=on
  Bus Selector : BusSelector  OutputSignals=VelocityX,VelocityY,VelocityZ
  Mux : Mux  Inputs=3
  animation mode : Subsystem
  elapsed track : Subsystem
  Out1 : Outport
  wires:
  animation mode/1(mode) -> Bus Creator/1  "Index"
  Bus Creator/1 -> Out1/1
  In1/1 -> Bus Selector/1
  elapsed track/1(s) -> Bus Creator/2  "Time"
  Bus Selector/3 -> Mux/3  "<VelocityZ>"
  Bus Selector/2 -> Mux/2  "<VelocityY>"
  Bus Selector/1 -> Mux/1  "<VelocityX>"
  Mux/1 -> animation mode/1(vel), elapsed track/1(vel)

== system example1_cs/Boy_150_1/SELF_Demux ==
  SELF : Inport  OutDataTypeStr=Bus: PRESCAN_SELFSENSORDATA
  Bus Selector : BusSelector  OutputSignals=PositionX,PositionY,PositionZ,OrientationRoll,OrientationPitch,OrientationYaw,Velocity,Yaw_rate,Lat,Long,Alt
  Demux2 : Demux  Outputs=3
  Gain : Gain  Gain=180/pi
  Gain1 : Gain  Gain=180/pi
  Vector Concatenate1 : Concatenate  NumInputs=3
  compas converter : Subsystem
  x [m] : Outport
  y [m] : Outport  Port=2
  z [m] : Outport  Port=3
  rotx [deg] : Outport  Port=4
  roty [deg] : Outport  Port=5
  rotz [deg] : Outport  Port=6
  GPS lat [deg] : Outport  Port=7
  GPS long [deg] : Outport  Port=8
  GPS alt [m] : Outport  Port=9
  velocity [m/s] : Outport  Port=10
  heading [deg] : Outport  Port=11
  yaw rate [deg/s] : Outport  Port=12
  wires:
  Bus Selector/11 -> GPS alt [m]/1  "<Alt>"
  Bus Selector/10 -> GPS long [deg]/1  "<Long>"
  Bus Selector/9 -> GPS lat [deg]/1  "<Lat>"
  Bus Selector/8 -> Gain1/1  "<Yaw_rate>"
  Bus Selector/7 -> velocity [m/s]/1  "<Velocity>"
  Bus Selector/6 -> compas converter/1(rotz [rad]), Vector Concatenate1/3  "<OrientationYaw>"
  Bus Selector/5 -> Vector Concatenate1/2  "<OrientationPitch>"
  Bus Selector/4 -> Vector Concatenate1/1  "<OrientationRoll>"
  Vector Concatenate1/1 -> Gain/1
  Bus Selector/3 -> z [m]/1  "<PositionZ>"
  Bus Selector/2 -> y [m]/1  "<PositionY>"
  Bus Selector/1 -> x [m]/1  "<PositionX>"
  SELF/1 -> Bus Selector/1
  Gain/1 -> Demux2/1
  Demux2/1 -> rotx [deg]/1
  Demux2/2 -> roty [deg]/1
  Demux2/3 -> rotz [deg]/1
  compas converter/1(heading [deg]) -> heading [deg]/1
  Gain1/1 -> yaw rate [deg/s]/1

== system example1_cs/Ford_Focus_Stationwagon_1/SELF_Demux ==
  SELF : Inport  OutDataTypeStr=Bus: PRESCAN_SELFSENSORDATA
  Bus Selector : BusSelector  OutputSignals=PositionX,PositionY,PositionZ,OrientationRoll,OrientationPitch,OrientationYaw,Velocity,Yaw_rate,Lat,Long,Alt
  Demux2 : Demux  Outputs=3
  Gain : Gain  Gain=180/pi
  Gain1 : Gain  Gain=180/pi
  Vector Concatenate1 : Concatenate  NumInputs=3
  compas converter : Subsystem
  x [m] : Outport
  y [m] : Outport  Port=2
  z [m] : Outport  Port=3
  rotx [deg] : Outport  Port=4
  roty [deg] : Outport  Port=5
  rotz [deg] : Outport  Port=6
  GPS lat [deg] : Outport  Port=7
  GPS long [deg] : Outport  Port=8
  GPS alt [m] : Outport  Port=9
  velocity [m/s] : Outport  Port=10
  heading [deg] : Outport  Port=11
  yaw rate [deg/s] : Outport  Port=12
  wires:
  Bus Selector/11 -> GPS alt [m]/1  "<Alt>"
  Bus Selector/10 -> GPS long [deg]/1  "<Long>"
  Bus Selector/9 -> GPS lat [deg]/1  "<Lat>"
  Bus Selector/8 -> Gain1/1  "<Yaw_rate>"
  Bus Selector/7 -> velocity [m/s]/1  "<Velocity>"
  Bus Selector/6 -> compas converter/1(rotz [rad]), Vector Concatenate1/3  "<OrientationYaw>"
  Bus Selector/5 -> Vector Concatenate1/2  "<OrientationPitch>"
  Bus Selector/4 -> Vector Concatenate1/1  "<OrientationRoll>"
  Vector Concatenate1/1 -> Gain/1
  Bus Selector/3 -> z [m]/1  "<PositionZ>"
  Bus Selector/2 -> y [m]/1  "<PositionY>"
  Bus Selector/1 -> x [m]/1  "<PositionX>"
  SELF/1 -> Bus Selector/1
  Gain/1 -> Demux2/1
  Demux2/1 -> rotx [deg]/1
  Demux2/2 -> roty [deg]/1
  Demux2/3 -> rotz [deg]/1
  compas converter/1(heading [deg]) -> heading [deg]/1
  Gain1/1 -> yaw rate [deg/s]/1

== system example1_cs/BMW_X5_SUV_1/BoundingRectangle_1_Demux/Signal2ArrayOfSignals1 ==
  note: Set mask parameter VECTORLENGTH
      |  to MAXMESSAGES
  note: Initial state of Previous vector block
      | set to zeros(VECTORLENGTH,1)
  LoopIndex : Inport
  Element : Inport  Port=2
  Assignment : Assignment  IndexOptions=Index vector (port)  Indices=1  OutputSizes=1
  Previous vector : Memory  InitialCondition=zeros(VECTORLENGTH,1)  InheritSampleTime=on
  ArrayofElements : Outport
  wires:
  Element/1 -> Assignment/2
  LoopIndex/1 -> Assignment/3
  Previous vector/1 -> Assignment/1
  Assignment/1 -> ArrayofElements/1, Previous vector/1

== system example1_cs/BMW_X5_SUV_1/BoundingRectangle_1_Demux/Signal2ArrayOfSignals2 ==
  note: Set mask parameter VECTORLENGTH
      |  to MAXMESSAGES
  note: Initial state of Previous vector block
      | set to zeros(VECTORLENGTH,1)
  LoopIndex : Inport
  Element : Inport  Port=2
  Assignment : Assignment  IndexOptions=Index vector (port)  Indices=1  OutputSizes=1
  Previous vector : Memory  InitialCondition=zeros(VECTORLENGTH,1)  InheritSampleTime=on
  ArrayofElements : Outport
  wires:
  Element/1 -> Assignment/2
  LoopIndex/1 -> Assignment/3
  Previous vector/1 -> Assignment/1
  Assignment/1 -> ArrayofElements/1, Previous vector/1
